simulink model "test_bench"  (R2016a)
settings: Solver=FixedStepAuto  StartTime=0.0  StopTime=inf  RelTol=1e-3
libraries: legoev3lib x8
settings Model: SimulationMode=external  ExtModeTrigDuration=2  Creator=Shobhit  LastModifiedBy=Shobhit
settings SolverCC: PositivePriorityOrder=on
settings OptimizationCC: OptimizeModelRefInitCode=on  LifeSpan=1  MaxStackSize=64
settings HardwareCC: ProdBitPerPointer=32  ProdLargestAtomicInteger=Long  ProdWordSize=32  ProdHWDeviceType=ARM Compatible->ARM 9  UseEmbeddedCoderFeatures=off  UseSimulinkCoderFeatures=off
settings RTWCC: SystemTargetFile=ert.tlc  HardwareBoard=LEGO MINDSTORMS EV3  TemplateMakefile=ert_default_tmf  GenerateReport=on  Toolchain=Sourcery G++ Lite v2009q3  IncludeHyperlinkInReport=on  LaunchReport=on  GenerateTraceInfo=on  GenerateTraceReport=on  GenerateTraceReportSl=on  GenerateTraceReportSf=on  GenerateTraceReportEml=on
settings CodeAppCC: ForceParamTrailComments=on  IgnoreCustomStorageClasses=off  OperatorAnnotations=on  SimulinkDataObjDesc=on  SFDataObjDesc=on  MATLABFcnDesc=on  MangleLength=10  InsertBlockDesc=on  MATLABSourceComments=on
settings ERTTargetCC: SupportContinuousTime=on  SupportNonInlinedSFcns=on  SupportVariableSizeSignals=on

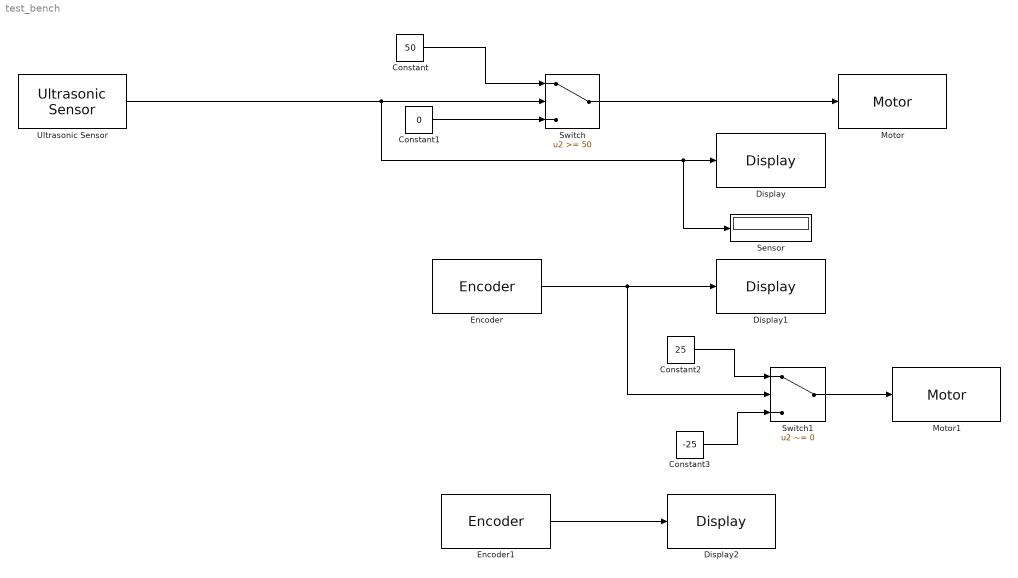
== system test_bench ==
  Constant : Constant  Value=50
  Constant1 : Constant  Value=0
  Constant2 : Constant  Value=25
  Constant3 : Constant  Value=-25
  Display : legoev3lib/Display  slcdStr=sensor  slcdLine=1  slcdFormat=Decimal
  Display1 : legoev3lib/Display  slcdStr=encA  slcdLine=2  slcdFormat=Decimal
  Display2 : legoev3lib/Display  slcdStr=encB  slcdLine=3  slcdFormat=Decimal
  Encoder : legoev3lib/Encoder  portNumber=A  opMode=Reset at each sample time  sampleTime=0.1
  Encoder1 : legoev3lib/Encoder  portNumber=B  opMode=Reset at each sample time  sampleTime=0.1
  Motor : legoev3lib/Motor  sportNumber=A  sstopAction=Brake
  Motor1 : legoev3lib/Motor  sportNumber=B  sstopAction=Brake
  Sensor : Display
  Switch : Switch  Threshold=50
  Switch1 : Switch  Criteria=u2 ~= 0  Threshold=50
  Ultrasonic Sensor : legoev3lib/Ultrasonic Sensor  PortNumber=1  sampleTime=0.1
  wires:
  Ultrasonic Sensor/1 -> Sensor/1, Display/1, Switch/2
  Switch/1 -> Motor/1
  Constant/1 -> Switch/1
  Constant1/1 -> Switch/3
  Encoder/1 -> Display1/1, Switch1/2
  Switch1/1 -> Motor1/1
  Constant2/1 -> Switch1/1
  Constant3/1 -> Switch1/3
  Encoder1/1 -> Display2/1
